simulink model "system1"  (R2023b)
settings: Solver=VariableStepAuto  StartTime=0.0  StopTime=10.0  RelTol=1e-3
undefined symbols (not defined in the file): b, c, d, x0
settings Model: Creator=roman  LastModifiedBy=roman

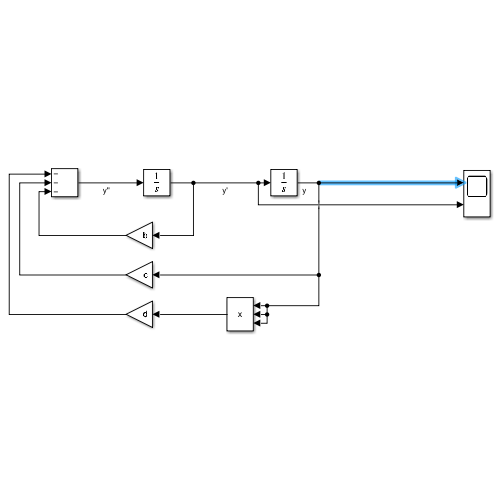
[thumbnail: Simulink's stored preview of the top-level diagram]
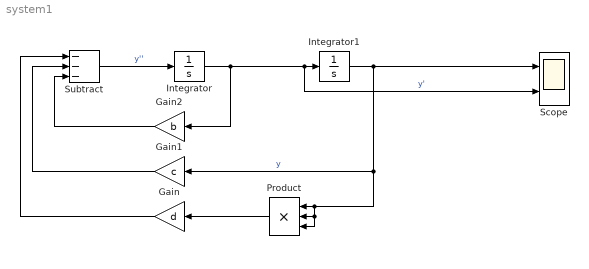
== system system1 ==
  Gain : Gain  Gain=d
  Gain1 : Gain  Gain=c
  Gain2 : Gain  Gain=b
  Integrator : Integrator  InitialCondition=x0(2)
  Integrator1 : Integrator  InitialCondition=x0(1)
  Product : Product  Inputs=3
  Scope : Scope  NumInputPorts=2
  Subtract : Sum  Inputs=---
  wires:
  Integrator/1 -> Gain2/1, Scope/2, Integrator1/1  "y'"
  Subtract/1 -> Integrator/1  "y''"
  Product/1 -> Gain/1
  Integrator1/1 -> Gain1/1, Product/2, Product/3, Product/1, Scope/1  "y"
  Gain/1 -> Subtract/1
  Gain1/1 -> Subtract/2
  Gain2/1 -> Subtract/3
